simulink model "test_controler"  (R2015a)
settings: Solver=FixedStepDiscrete  StartTime=0.0  StopTime=10.0  RelTol=1e-3
values from neighbouring files (symbols this model uses):
  Nbar = Nu+K*Nx    [compute_gain.m]    (also in end_of_class.mat = 0.700435596375; log_observer_test.mat = 0.700435596375)
  T = 0.02    [end_of_class.mat]    (also in gera_signals.m; log_observer_test.mat)
settings Model: Creator=alunos  LastModifiedBy=hdplsa
settings DataIOCC: LimitDataPoints=off

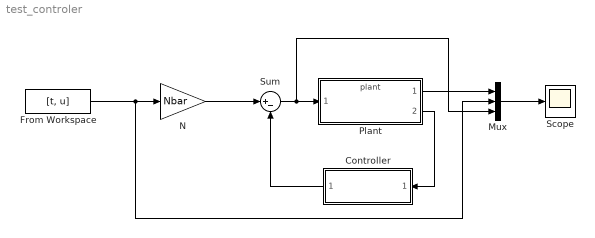
== system test_controler ==
  Controller : ModelReference  ModelNameDialog=controller.slx  SimulationMode=Normal  ModelReferenceVersion=1.2  CopyOfModelName=controller.slx  DefaultDataLogging=on
  From Workspace : FromWorkspace  VariableName=[t, u]  SampleTime=T
  Mux : Mux  Inputs=3
  N : Gain  Gain=Nbar
  Plant : ModelReference  ModelNameDialog=plant.slx  SimulationMode=Normal  ModelReferenceVersion=1.2  CopyOfModelName=plant.slx  DefaultDataLogging=on
  Scope : Scope
      settings: SaveName=test_controller
  Sum : Sum  Inputs=|+-
  wires:
  From Workspace/1 -> Mux/2, N/1
  N/1 -> Sum/1
  Controller/1 -> Sum/2
  Plant/1 -> Mux/1
  Mux/1 -> Scope/1
  Plant/2 -> Controller/1
  Sum/1 -> Mux/3, Plant/1
